simulink model "ELEC522_PROJECT2"  (Simulink 8.9)
settings: Solver=VariableStepAuto  StartTime=0.0  StopTime=10  RelTol=1e-3
undefined symbols (not defined in the file): A, N
libraries: xbsIndex_r4 x127, JTAGRuntimeCosim_r4 x1
(part 2 of 2)

== system ELEC522_PROJECT2/Matrix Multiplication module/PE: MAC8 ==
  B : Inport
  A : Inport  Port=2
  reset : Inport  Port=3
  pre_input : Inport  Port=4
  Accumulator : xbsIndex_r4/Accumulator  operation=Add  n_bits=28  overflow=Wrap  scale=1  rst=on  hasbypass=off  infoeditControl=reset for floating point data type must be asserted for a minimum of 2 cycles  en=off  latency=1  msb_inp=100  msb=100  lsb=-100  use_behavioral_HDL=on  implementation=Fabric  dbl_ovrd=off  block_type=accum
  Constant : xbsIndex_r4/Constant  const=1.0  gui_display_data_type=Boolean  arith_type=Boolean  n_bits=16  bin_pt=14  preci_type=Single  exp_width=8  frac_width=24  explicit_period=on  period=1  equ=P=C  opselect=C  inp2=PCIN>>17  opr=+  inp1=P  carry=CIN  dbl_ovrd=off  block_type=constant
  Delay : xbsIndex_r4/Delay  rst=off  infoeditControl=Selection of Reset will increase slice count due to use of real FFs and instead of SRLs  en=off  latency=1  reg_retiming=off  dbl_ovrd=off  block_type=delay
  Delay1 : xbsIndex_r4/Delay  rst=off  infoeditControl=Selection of Reset will increase slice count due to use of real FFs and instead of SRLs  en=off  latency=1  reg_retiming=off  dbl_ovrd=off  block_type=delay
  Delay2 : xbsIndex_r4/Delay  rst=off  infoeditControl=Selection of Reset will increase slice count due to use of real FFs and instead of SRLs  en=off  latency=9  reg_retiming=off  dbl_ovrd=off  block_type=delay
  Mult : xbsIndex_r4/Mult  precision=Full  arith_type="Signed  (2's comp)"  n_bits=16  bin_pt=14  quantization=Truncate  overflow=Wrap  en=off  latency=0  use_behavioral_HDL=off  opt=Speed  use_embedded=on  optimum_pipeline=off  pipeline=on  dbl_ovrd=off  use_rpm=on  placement_style=Triangular  block_type=mult
  Mux : xbsIndex_r4/Mux  inputs=2  en=off  latency=0  precision=Full  arith_type=Unsigned  n_bits=16  bin_pt=14  quantization=Truncate  overflow=Wrap  dbl_ovrd=off  block_type=mux
  B1 : Outport
  A1 : Outport  Port=2
  C1 : Outport  Port=3
  wires:
  A/1 -> Delay1/1, Mult/2
  B/1 -> Delay/1, Mult/1
  Mult/1 -> Accumulator/1
  Delay1/1 -> A1/1
  Delay/1 -> B1/1
  reset/1 -> Accumulator/2
  Accumulator/1 -> Mux/2
  Mux/1 -> C1/1
  Constant/1 -> Delay2/1
  Delay2/1 -> Mux/1
  pre_input/1 -> Mux/3

== system ELEC522_PROJECT2/Matrix Multiplication module/PE: MAC9 ==
  B : Inport
  A : Inport  Port=2
  reset : Inport  Port=3
  Accumulator : xbsIndex_r4/Accumulator  operation=Add  n_bits=28  overflow=Wrap  scale=1  rst=on  hasbypass=off  infoeditControl=reset for floating point data type must be asserted for a minimum of 2 cycles  en=off  latency=1  msb_inp=100  msb=100  lsb=-100  use_behavioral_HDL=on  implementation=Fabric  dbl_ovrd=off  block_type=accum
  Delay1 : xbsIndex_r4/Delay  rst=off  infoeditControl=Selection of Reset will increase slice count due to use of real FFs and instead of SRLs  en=off  latency=1  reg_retiming=off  dbl_ovrd=off  block_type=delay
  Mult : xbsIndex_r4/Mult  precision=Full  arith_type="Signed  (2's comp)"  n_bits=16  bin_pt=14  quantization=Truncate  overflow=Wrap  en=off  latency=0  use_behavioral_HDL=off  opt=Speed  use_embedded=on  optimum_pipeline=off  pipeline=on  dbl_ovrd=off  use_rpm=on  placement_style=Triangular  block_type=mult
  C1 : Outport
  A2 : Outport  Port=2
  wires:
  A/1 -> Delay1/1, Mult/2
  B/1 -> Mult/1
  Mult/1 -> Accumulator/1
  Delay1/1 -> A2/1
  reset/1 -> Accumulator/2
  Accumulator/1 -> C1/1

== matlab function adjust output matrix /MATLAB Function1 ==
  data: c1 input double; y output double; c2 input double; c3 input double; c4 input double
function y = fcn(c1,c2,c3,c4)
u=[c1';c2';c3';c4'];
y = u;
